simulink model "Q2_3_sim"  (R2015b)
settings: Solver=VariableStepAuto  StartTime=0.0  StopTime=30  RelTol=1e-3
values from neighbouring files (symbols this model uses):
  F = 24    [Q2_3.m]
  M_T = m_s + m_r + 2*m_p + m_f    (= 121.07)    [Q2_3.m]
settings Model: Creator=SooJengTan  LastModifiedBy=SooJengTan

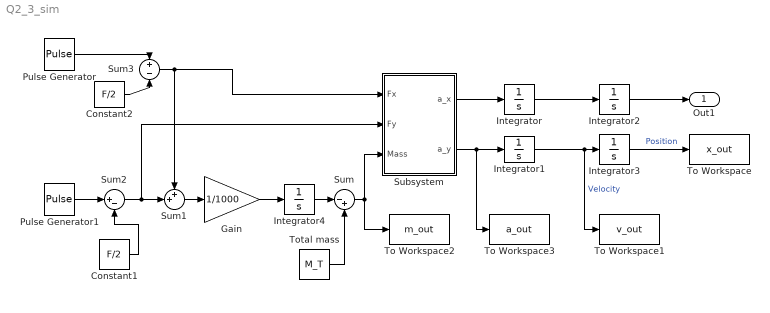
== system Q2_3_sim ==
  Constant1 : Constant  Value=F/2
  Constant2 : Constant  Value=F/2
  Gain : Gain  Gain=1/1000
  Integrator{,1..4} (5 alike) : Integrator
  Pulse Generator : DiscretePulseGenerator  PulseType=Time based  Amplitude=F  Period=20  PulseWidth=50
  Pulse Generator1 : DiscretePulseGenerator  PulseType=Time based  Amplitude=F  Period=20  PulseWidth=50
  Subsystem : Subsystem
  Sum : Sum  Inputs=|-+
  Sum1 : Sum  Inputs=++|
  Sum2 : Sum  Inputs=|+-
  Sum3 : Sum  Inputs=+-
  To Workspace : ToWorkspace  VariableName=x_out  SaveFormat=Structure With Time  SampleTime=-1
  To Workspace1 : ToWorkspace  VariableName=v_out  SaveFormat=Structure With Time  SampleTime=-1
  To Workspace2 : ToWorkspace  VariableName=m_out  SaveFormat=Structure With Time  SampleTime=-1
  To Workspace3 : ToWorkspace  VariableName=a_out  SaveFormat=Structure With Time  SampleTime=-1
  Total mass : Constant  Value=M_T
  Out1 : Outport
  wires:
  Subsystem/1(a_x) -> Integrator/1
  Subsystem/2(a_y) -> To Workspace3/1, Integrator1/1
  Integrator/1 -> Integrator2/1
  Integrator1/1 -> To Workspace1/1, Integrator3/1  "Velocity"
  Integrator3/1 -> To Workspace/1  "Position"
  Integrator2/1 -> Out1/1
  Gain/1 -> Integrator4/1
  Integrator4/1 -> Sum/1
  Total mass/1 -> Sum/2
  Sum1/1 -> Gain/1
  Sum/1 -> To Workspace2/1, Subsystem/3(Mass)
  Constant1/1 -> Sum2/2
  Pulse Generator1/1 -> Sum2/1
  Sum2/1 -> Sum1/2, Subsystem/2(Fy)
  Pulse Generator/1 -> Sum3/1
  Constant2/1 -> Sum3/2
  Sum3/1 -> Sum1/1, Subsystem/1(Fx)

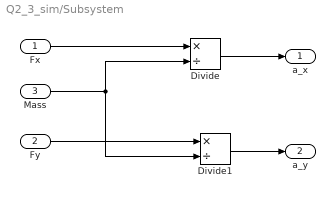
== system Q2_3_sim/Subsystem ==
  Fx : Inport
  Fy : Inport  Port=2
  Mass : Inport  Port=3
  Divide : Product  Inputs=*/
  Divide1 : Product  Inputs=*/
  a_x : Outport
  a_y : Outport  Port=2
  wires:
  Fx/1 -> Divide/1
  Mass/1 -> Divide/2, Divide1/2
  Divide/1 -> a_x/1
  Divide1/1 -> a_y/1
  Fy/1 -> Divide1/1
